simulink model "mod1"  (Simulink 8.1)
settings: Solver=FixedStepDiscrete  StartTime=0.0  StopTime=10e-3  RelTol=1e-3
undefined symbols (not defined in the file): Fs, modctrl
libraries: dspsigops x2, dspsrcs4 x1
settings Model: Creator=amyles  LastModifiedBy=amyles
settings DataIOCC: LimitDataPoints=off  MaxDataPoints=50000
settings OptimizationCC: InlineParams=on
settings DebuggingCC: StrictBusMsg=Warning
settings ModelReferenceCC: ModelReferenceNumInstancesAllowed=Single

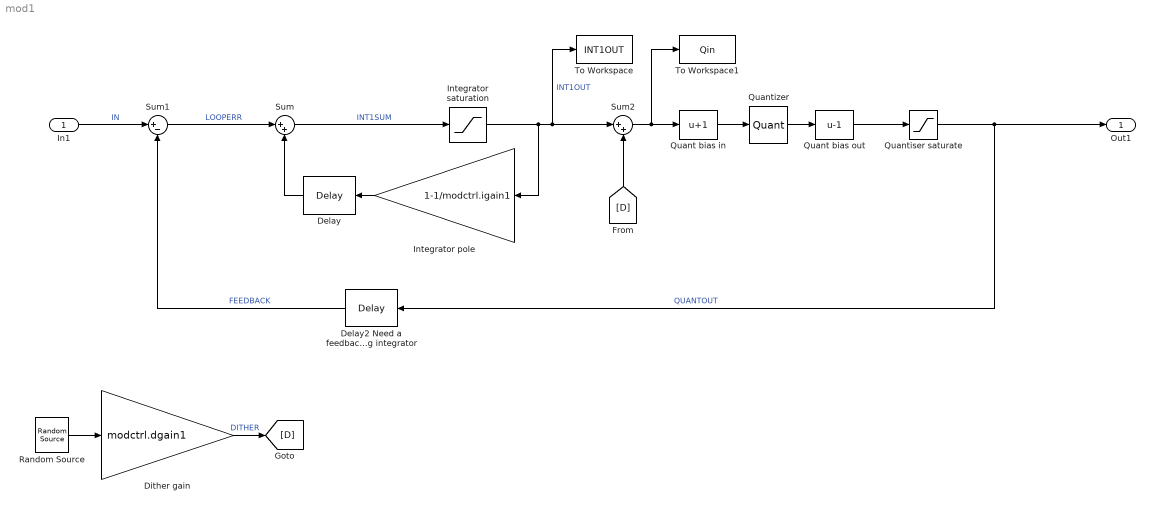
== system mod1 ==
  In1 : Inport
  Delay : dspsigops/Delay  InputProcessing=Inherited (this choice will be removed - see release notes)  dly_unit=Samples  delay=1  ic_detail=off  dif_ic_for_ch=off  dif_ic_for_dly=off  ic=0  reset_popup=None
  Delay2 Need a feedback delay to avoid a delay-free loop as we had a non-delaying integrator : dspsigops/Delay  InputProcessing=Inherited (this choice will be removed - see release notes)  dly_unit=Samples  delay=1  ic_detail=off  dif_ic_for_ch=off  dif_ic_for_dly=off  ic=0  reset_popup=None
  Dither gain : Gain  Gain=modctrl.dgain1
      settings: AttributesFormatString=Dither level adjust
  Integrator pole : Gain  Gain=1-1/modctrl.igain1
      settings: AttributesFormatString=(model finite dc gain)
  Integrator saturation : Saturate  UpperLimit=modctrl.isat1  LowerLimit=-(modctrl.isat1)
  Quant bias in : Bias  Bias=1
      settings: AttributesFormatString=Need offset to give\nMID-RISE quantiser
  Quant bias out : Bias  Bias=-1
      settings: AttributesFormatString=Shift outputs to\n..., -2, 1, 1, ...
  Quantiser saturate : Saturate  UpperLimit=1  LowerLimit=-1
      settings: AttributesFormatString=Limit quantiser\noutput to +/-1
  Quantizer : Quantizer  QuantizationInterval=2  LinearizeAsGain=off
      settings: AttributesFormatString=step = 2
  Random Source : dspsrcs4/Random Source  SrcType=Uniform  NormMethod=Ziggurat  CltLength=12  MinVal=-1  MaxVal=1  MeanVal=0  VarVal=1  RepMode=Not repeatable  rawSeed=1  IsInherit=off  SampMode=Discrete  SampTime=1/Fs  SampFrame=1  DataType=Double  OutComplex=Real
      settings: AttributesFormatString=Dither source
  Sum : Sum  Inputs=|++
      settings: AttributesFormatString=Integrator summer
  Sum1 : Sum  Inputs=|+-
      settings: AttributesFormatString=Modulator input\nloop servo error (input - fbk)
  Sum2 : Sum  Inputs=|++
  To Workspace : ToWorkspace  VariableName=INT1OUT  SampleTime=-1
  To Workspace1 : ToWorkspace  VariableName=Qin  SampleTime=-1
  Out1 : Outport
  wires:
  Delay/1 -> Sum/2
  Sum/1 -> Integrator saturation/1  "INT1SUM"
  Sum1/1 -> Sum/1  "LOOPERR"
  Delay2 Need a feedback delay to avoid a delay-free loop as we had a non-delaying integrator/1 -> Sum1/2  "FEEDBACK"
  In1/1 -> Sum1/1  "IN"
  Quant bias in/1 -> Quantizer/1
  Sum2/1 -> Quant bias in/1, To Workspace1/1
  Integrator pole/1 -> Delay/1
  Quantiser saturate/1 -> Delay2 Need a feedback delay to avoid a delay-free loop as we had a non-delaying integrator/1, Out1/1  "QUANTOUT"
  Quantizer/1 -> Quant bias out/1
  Quant bias out/1 -> Quantiser saturate/1
  Integrator saturation/1 -> Integrator pole/1, Sum2/1, To Workspace/1  "INT1OUT"
  Random Source/1 -> Dither gain/1
  Dither gain/1 -> [D]  "DITHER"
  [D] -> Sum2/2
